simulink model "Project1_Part2"  (R2023b)
settings: Solver=ode1  StartTime=0.0  StopTime=25  FixedStep=.1  RelTol=1e-3
values from neighbouring files (symbols this model uses):
  A_var = A(i)    [Project1_Part2_matlab.m]    (also in init.m = 0; plotting_loop.m = 100)
  b1_var = 1    [Project1_Part2_matlab.m]
  b2_var = 1    [Project1_Part2_matlab.m]
  J1_var = 100    [Project1_Part2_matlab.m]
  J2_var = 1    [Project1_Part2_matlab.m]
settings Model: Creator=turtl  LastModifiedBy=rahma

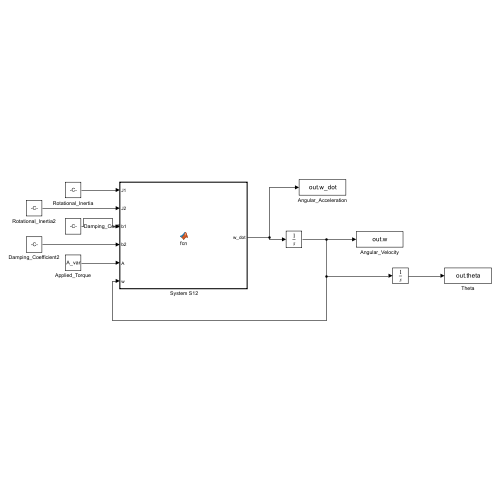
[thumbnail: Simulink's stored preview of the top-level diagram]
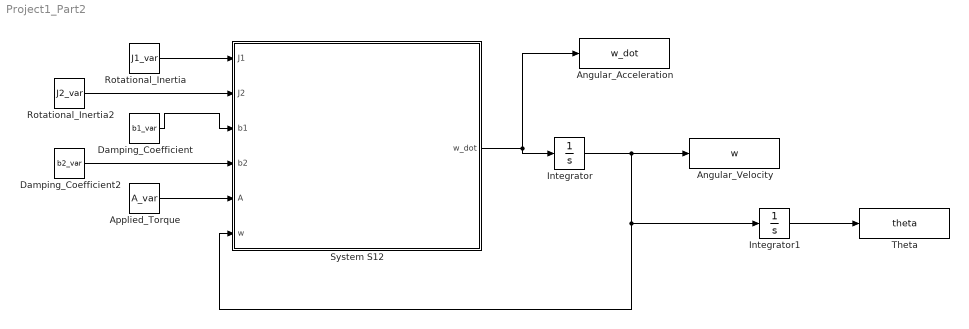
== system Project1_Part2 ==
  " System S12" : MATLAB Function  TreatAsAtomicUnit=on
  Angular_Acceleration : ToWorkspace  VariableName=w_dot  SaveFormat=Timeseries  SampleTime=-1
  Angular_Velocity : ToWorkspace  VariableName=w  SaveFormat=Timeseries  SampleTime=-1
  Applied_Torque : Constant  Value=A_var
  Damping_Coefficient : Constant  Value=b1_var
  Damping_Coefficient2 : Constant  Value=b2_var
  Integrator : Integrator  UpperSaturationLimit=10000  LowerSaturationLimit=0
  Integrator1 : Integrator
  Rotational_Inertia : Constant  Value=J1_var
  Rotational_Inertia2 : Constant  Value=J2_var
  Theta : ToWorkspace  VariableName=theta  SaveFormat=Timeseries  SampleTime=-1
  wires:
  Applied_Torque/1 -> " System S12"/5(A)
  Integrator/1 -> Angular_Velocity/1, Integrator1/1, " System S12"/6(w)
  Damping_Coefficient/1 -> " System S12"/3(b1)
  Rotational_Inertia/1 -> " System S12"/1(J1)
  Integrator1/1 -> Theta/1
  " System S12"/1(w_dot) -> Angular_Acceleration/1, Integrator/1
  Rotational_Inertia2/1 -> " System S12"/2(J2)
  Damping_Coefficient2/1 -> " System S12"/4(b2)

== matlab function Project1_Part2/ System S12 ==
  data: J1 input; w_dot output; J2 input; b1 input; b2 input; A input; w input
function w_dot = fcn(J1,J2, b1,b2, A,w)

tau_damped = (b1*w)-(b2*w);
w_dot = (1/(J1+J2))*(A-tau_damped);

end
